simulink model "weixing3_pd_ekf"  (R2019a)
settings: Solver=FixedStepAuto  StartTime=0.0  StopTime=40  FixedStep=0.001  RelTol=1e-3  EnableMultiTasking=on
values from neighbouring files (symbols this model uses):
  f = Jn\M(:,i)    [Copy_of_flexcont_Slidemode.m]    (also in flash.m = getframe(gcf); flexcont1_wb.m = -H'*wv(:,i); flexcont2.m; flexcont2_wb.m)
libraries: instrumentlib x2, simulink x1
settings Model: Creator=Administrator  LastModifiedBy=HP
settings DataIOCC: ExternalInput=[t, y]  LimitDataPoints=on  MaxDataPoints=15000  ReturnWorkspaceOutputs=off
settings OptimizationCC: LifeSpan=inf
settings DebuggingCC: MultiTaskCondExecSysMsg=warning  MultiTaskRateTransMsg=warning  AllowSymbolicDim=off  SFUnexpectedBacktrackingDiag=warning  SFNoUnconditionalDefaultTransitionDiag=warning  SFExecutionAtInitializationDiag=none  ArithmeticOperatorsInVariantConditions=warning
settings ModelReferenceCC: PropagateSignalLabelsOutOfModel=off
settings SFSimCC: SimUseLocalCustomCode=off
settings RTWCC: RTWUseLocalCustomCode=off
settings CodeAppCC: StateflowObjectComments=on
settings GRTTargetCC: TargetLangStandard=C89/C90 (ANSI)
settings ConfigComp: CovMetricSettings=dw  CovHtmlReporting=on  CovSaveCumulativeToWorkspaceVar=on  CovSaveSingleToWorkspaceVar=on  CovExternalEMLEnable=off

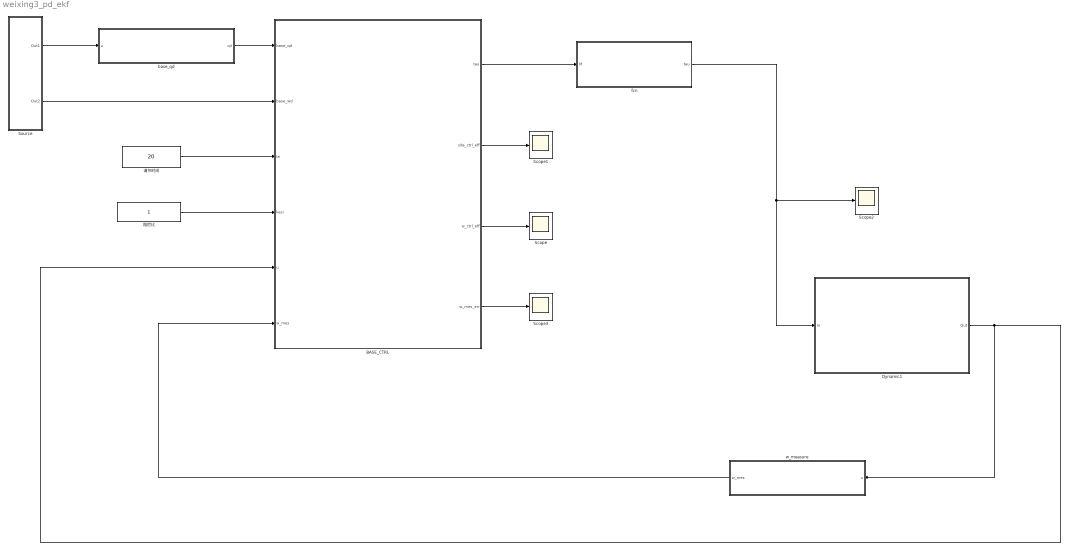
== system weixing3_pd_ekf ==
  " Dynamic1" : Subsystem  Description=|  mask{com_step=0.001, tcp_data_size=16, host_name=localhost, tcp_port=50028, tcp_timeout=15}
      | This block can be used to exchange data with Chrono::Engine.                                                                                      
      | A Chrono::Engine program with a running ChCosimulation inferface must be started, it will work as a server; then the Simulink program must be run.
      | Note! check that the dimensions of the exchanged vectors do match!
      mask prompts: com_step "Communication step size"; tcp_data_size "N. of scalars received from C::E (as block output)"; host_name "TCP host name (ex. 'localhost', or 'www.myhost.com')"; tcp_port "TCP port (ex. 50007)"; tcp_timeout "TCP timeout (seconds)"
      mask init:
      | block_receive = [gcb, '/TCP Receive'];
      | set_param(block_receive, 'SampleTime', num2str(com_step));
      | set_param(block_receive, 'Host', host_name);
      | set_param(block_receive, 'Port', num2str(tcp_port));
      | set_param(block_receive, 'DataSize', num2str(tcp_data_size));
      | set_param(block_receive, 'Timeout', num2str(tcp_timeout));
      | block_send = [gcb, '/TCP Send'];
      | set_param(block_send, 'Host', host_name);
      | set_param(block_send, 'Port', num2str(tcp_port));
      mask Display: disp('MBSim CoSim/Matlab')
  BASE_CTRL : MATLAB Function  TreatAsAtomicUnit=on
  Scope{,1..3} (4 alike) : Scope
  Source : Subsystem
  base_qd : MATLAB Function  TreatAsAtomicUnit=on
  fcn : MATLAB Function  TreatAsAtomicUnit=on
  w_measure : MATLAB Function  TreatAsAtomicUnit=on
  调节时间 : Constant  Value=20
  阻尼比 : Constant
  wires:
  base_qd/1(q4) -> BASE_CTRL/1(base_qd)
  Source/2(Out2) -> BASE_CTRL/2(base_wd)
  调节时间/1 -> BASE_CTRL/3(tn)
  阻尼比/1 -> BASE_CTRL/4(kesi)
  BASE_CTRL/3(w_ctrl_eff) -> Scope/1
  BASE_CTRL/2(sita_ctrl_eff) -> Scope1/1
  " Dynamic1"/1(Out) -> w_measure/1(u), BASE_CTRL/5(u)
  Source/1(Out1) -> base_qd/1(u)
  BASE_CTRL/1(tau) -> fcn/1(M)
  fcn/1(tau) -> Scope2/1, " Dynamic1"/1(In)
  BASE_CTRL/4(w_mes_err) -> Scope3/1
  w_measure/1(w_mes) -> BASE_CTRL/6(w_mes)

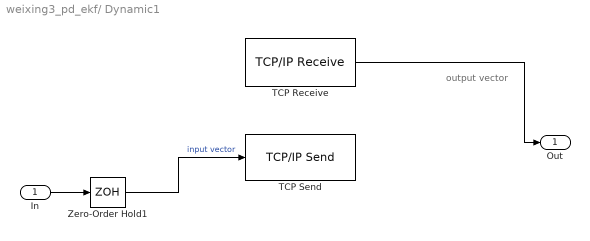
== system weixing3_pd_ekf/ Dynamic1 ==
  note: output vector
  In : Inport
  TCP Receive : instrumentlib/TCP//IP Receive  Priority=1  Host=localhost  Port=50028  DataSize=16  EnableBlockingMode=on  Timeout=15  SampleTime=0.001  DataType=double  ByteOrder=LittleEndian  ASCIIFormatting=%f,  Terminator=LF
      settings: SourceProductName=Instrument Control Toolbox
  TCP Send : instrumentlib/TCP//IP Send  Priority=2  Host=localhost  Port=50028  EnableBlockingMode=off  Timeout=10  ByteOrder=LittleEndian  TransferDelay=on
      settings: SourceProductName=Instrument Control Toolbox
  Zero-Order Hold1 : ZeroOrderHold  SampleTime=com_step
  Out : Outport
  wires:
  Zero-Order Hold1/1 -> TCP Send/1  "input vector"
  In/1 -> Zero-Order Hold1/1
  TCP Receive/1 -> Out/1

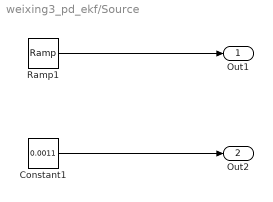
== system weixing3_pd_ekf/Source ==
  Constant1 : Constant  Value=0.0011
  Ramp1 : simulink/Sources/Ramp  slope=0.0011  start=0  InitialOutput=0
  Out1 : Outport
  Out2 : Outport  Port=2
  wires:
  Constant1/1 -> Out2/1
  Ramp1/1 -> Out1/1

== matlab function weixing3_pd_ekf/base_qd ==
  data: u input; q4 output
function q4 = fcn(u)
    base_qd=zeros(4,1);
    base_qd(1)=cos(u/2);
    base_qd(2)=sin(u/2);
    q1=[cos(-10*pi/180/2);0;sin(-10*pi/180/2);0];
    q2=[cos(-10*pi/180/2);sin(-10*pi/180/2);0;0];
    q3=[q1(1) -q1(2) -q1(3) -q1(4);
    q1(2) q1(1) -q1(4) q1(3);
    q1(3) q1(4) q1(1) -q1(2);
    q1(4) -q1(3) q1(2) q1(1)]*q2;
    q4=[q3(1) -q3(2) -q3(3) -q3(4);
    q3(2) q3(1) -q3(4) q3(3);
    q3(3) q3(4) q3(1) -q3(2);
    q3(4) -q3(3) q3(2) q3(1)]*base_qd;
end

== matlab function weixing3_pd_ekf/w_measure ==
  data: u input; w_mes output
function w_mes = fcn(u)
base_q=u(6:9);
base_qv=u(13:16);
w=2*[-base_q(2),base_q(1),base_q(4),-base_q(3);
    -base_q(3),-base_q(4),base_q(1),base_q(2);
    -base_q(4),base_q(3),-base_q(2),base_q(1)]*base_qv;
noise_mes=5.8178e-04;%1sigm  0.1deg/s(3sigm)
w_mes=w+noise_mes*randn(3,1);
end

== matlab function weixing3_pd_ekf/BASE_CTRL ==
  data: tau output; sita_ctrl_eff output; w_ctrl_eff output; base_qd input; base_wd input; tn input; kesi input; u input; w_mes input; w_mes_err output
function [tau,sita_ctrl_eff,w_ctrl_eff,w_mes_err]  =fcn(base_qd,base_wd,tn,kesi,u,w_mes)
%%%%%MBSim输出信息
time=u(1);
time_step=u(2);
base_p=u(3:5);
base_q=u(6:9);
base_pv=u(10:12);
base_qv=u(13:16);

% %测量星体角速度（在本体系下）/滤波得到
w=w_mes;

%构造角速度叉乘矩阵
W=[0 -w(3) w(2);w(3) 0 -w(1);-w(2) w(1) 0];
%四元数误差
qe=[base_qd(1),base_qd(2),base_qd(3),base_qd(4);
    -base_qd(2),base_qd(1),base_qd(4),-base_qd(3);
    -base_qd(3),-base_qd(4),base_qd(1),base_qd(2);
    -base_qd(4),base_qd(3),-base_qd(2),base_qd(1)]*base_q;
%取矢量部分
qe1=qe(2:4);
%期望的姿态变换矩阵
A_OBd=[1-2*base_qd(3)^2-2*base_qd(4)^2,2*(base_qd(2)*base_qd(3)-base_qd(1)*base_qd(4)),2*(base_qd(2)*base_qd(4)+base_qd(1)*base_qd(3));
    2*(base_qd(2)*base_qd(3)+base_qd(1)*base_qd(4)),1-2*base_qd(2)^2-2*base_qd(4)^2,2*(base_qd(4)*base_qd(3)-base_qd(1)*base_qd(2));
    2*(base_qd(2)*base_qd(4)-base_qd(1)*base_qd(3)),2*(base_qd(4)*base_qd(3)+base_qd(1)*base_qd(2)),1-2*base_qd(2)^2-2*base_qd(3)^2];
%实际的基体姿态变换矩阵(相对于惯性坐标系)
A_OB=[1-2*base_q(3)^2-2*base_q(4)^2,2*(base_q(2)*base_q(3)-base_q(1)*base_q(4)),2*(base_q(2)*base_q(4)+base_q(1)*base_q(3));
    2*(base_q(2)*base_q(3)+base_q(1)*base_q(4)),1-2*base_q(2)^2-2*base_q(4)^2,2*(base_q(4)*base_q(3)-base_q(1)*base_q(2));
    2*(base_q(2)*base_q(4)-base_q(1)*base_q(3)),2*(base_q(4)*base_q(3)+base_q(1)*base_q(2)),1-2*base_q(2)^2-2*base_q(3)^2];
A_dB=A_OBd\A_OB;%(由误差四元数构成的姿态变换矩阵)
%角速率误差
we=w-[base_wd;0;0];

% %计算固有频率
wn=10/(kesi*tn);
%%%%%%%%%%%%%%控制率设计
%参数选取与计算
k=wn^2*2;
d=2*kesi*wn;
Jn=[566.7165 -3.77077 -3.77077;-3.77077 3658.9667 -3.77077;-3.77077 -3.77077 3705.628];
D=d*Jn;
K4=k*Jn;
%控制率
tau=zeros(3,1);
tau(1:3)=W*Jn*w-K4*qe1-D*we;

%输出指标-欧拉角误差
%根据本体和期望之间的姿态变换矩阵求解欧拉角
sita_ze=atan(-A_dB(1,2)/A_dB(1,1));
sita_ye=asin(A_dB(1,3));
sita_xe=-asin(A_dB(2,3)/cos(sita_ye));
%输出角度单位
sita_ctrl_eff=[sita_xe;sita_ye;sita_ze]*180/pi;
%输出指标-角速度
w_actual=2*[-base_q(2),base_q(1),base_q(4),-base_q(3);
    -base_q(3),-base_q(4),base_q(1),base_q(2);
    -base_q(4),base_q(3),-base_q(2),base_q(1)]*base_qv;
w_ctrl_eff=[w_actual;[base_wd;0;0]]*180/pi;
%输出指标-测量误差
w_mes_err=(w-w_actual)*180/pi;

end

== matlab function weixing3_pd_ekf/fcn ==
  data: M input; tau output
function tau = fcn(M)


tau=[M(1);M(2);M(3);zeros(6,1);1];
end
